simulink model "Computed_Impedance"  (R2023b)
settings: Solver=VariableStepAuto  StartTime=0.0  StopTime=10.0  RelTol=1e-3
settings Model: Creator=91996  LastModifiedBy=91996

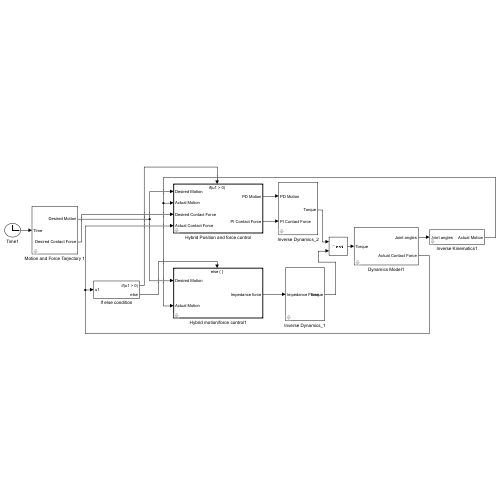
[thumbnail: Simulink's stored preview of the top-level diagram]
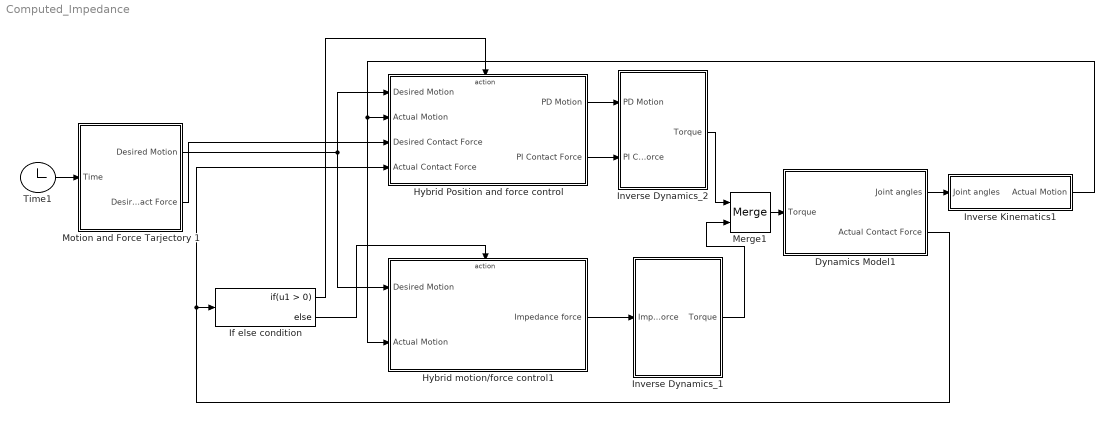
== system Computed_Impedance ==
  Dynamics Model1 : Subsystem
      mask DialogControl C Prompt: Parameters
  Hybrid Position and force control : Subsystem
      mask DialogControl A Prompt: Parameters
  Hybrid motion/force control1 : Subsystem
      mask DialogControl A Prompt: Parameters
  If else condition : If
  Inverse Dynamics_1 : Subsystem
      mask DialogControl B Prompt: Parameters
  Inverse Dynamics_2 : Subsystem
      mask DialogControl B Prompt: Parameters
  Inverse Kinematics1 : Subsystem
      mask DialogControl Kinematics Prompt: Parameters
  Merge1 : Merge
  Motion and Force Tarjectory 1 : Subsystem
      mask DialogControl E Prompt: Parameters
  Time1 : Clock
  wires:
  If else condition/2 -> Hybrid motion/force control1/Action
  Merge1/1 -> Dynamics Model1/1(Torque)
  Time1/1 -> Motion and Force Tarjectory 1/1(Time)
  Inverse Dynamics_1/1(Torque) -> Merge1/2
  Inverse Dynamics_2/1(Torque) -> Merge1/1
  Dynamics Model1/2(Actual Contact Force) -> If else condition/1, Hybrid Position and force control/4(Actual Contact Force)
  Hybrid Position and force control/2(PI Contact Force) -> Inverse Dynamics_2/2(PI Contact Force)
  Motion and Force Tarjectory 1/2(Desired Contact Force) -> Hybrid Position and force control/3(Desired Contact Force)
  If else condition/1 -> Hybrid Position and force control/Action
  Motion and Force Tarjectory 1/1(Desired Motion) -> Hybrid motion/force control1/1(Desired Motion), Hybrid Position and force control/1(Desired Motion)
  Hybrid motion/force control1/1(Impedance force) -> Inverse Dynamics_1/1(Impedance Force)
  Dynamics Model1/1(Joint angles) -> Inverse Kinematics1/1(Joint angles)
  Hybrid Position and force control/1(PD Motion) -> Inverse Dynamics_2/1(PD Motion)
  Inverse Kinematics1/1(Actual Motion) -> Hybrid motion/force control1/2(Actual Motion), Hybrid Position and force control/2(Actual Motion)

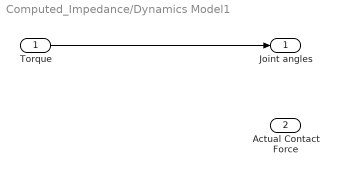
== system Computed_Impedance/Dynamics Model1 ==
  Torque : Inport
  Joint angles : Outport
  Actual Contact Force : Outport  Port=2
  wires:
  Torque/1 -> Joint angles/1

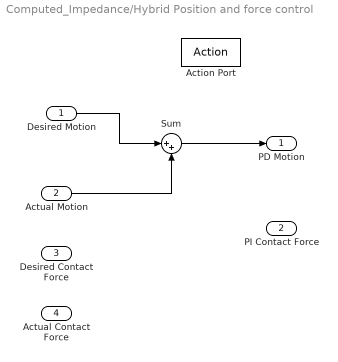
== system Computed_Impedance/Hybrid Position and force control ==
  Desired Motion : Inport
  Actual Motion : Inport  Port=2
  Desired Contact Force : Inport  Port=3
  Actual Contact Force : Inport  Port=4
  Action Port : ActionPort  ActionPortLabel=if(u1 > 0)
  Sum : Sum  Inputs=|++
  PD Motion : Outport
  PI Contact Force : Outport  Port=2
  wires:
  Desired Motion/1 -> Sum/1
  Actual Motion/1 -> Sum/2
  Sum/1 -> PD Motion/1

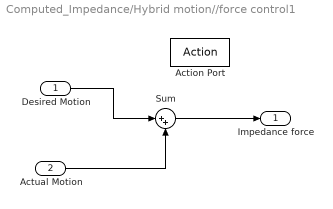
== system Computed_Impedance/Hybrid motion//force control1 ==
  Desired Motion : Inport
  Actual Motion : Inport  Port=2
  Action Port : ActionPort  ActionPortLabel=else
  Sum : Sum  Inputs=|++
  Impedance force : Outport
  wires:
  Desired Motion/1 -> Sum/1
  Actual Motion/1 -> Sum/2
  Sum/1 -> Impedance force/1

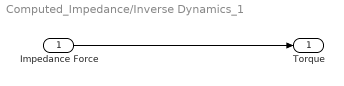
== system Computed_Impedance/Inverse Dynamics_1 ==
  Impedance Force : Inport
  Torque : Outport
  wires:
  Impedance Force/1 -> Torque/1

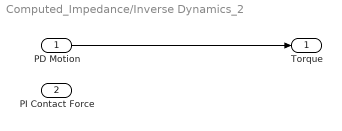
== system Computed_Impedance/Inverse Dynamics_2 ==
  PD Motion : Inport
  PI Contact Force : Inport  Port=2
  Torque : Outport
  wires:
  PD Motion/1 -> Torque/1

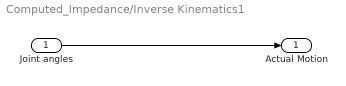
== system Computed_Impedance/Inverse Kinematics1 ==
  Joint angles : Inport
  Actual Motion : Outport
  wires:
  Joint angles/1 -> Actual Motion/1

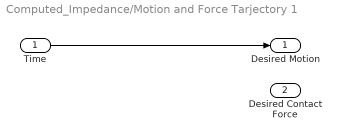
== system Computed_Impedance/Motion and Force Tarjectory 1 ==
  Time : Inport
  Desired Motion : Outport
  Desired Contact Force : Outport  Port=2
  wires:
  Time/1 -> Desired Motion/1
